simulink model "Sim_Riementrieb"  (R2015b)
settings: Solver=ode45  SolverMode=SingleTasking  StartTime=0.0  StopTime=10.0  RelTol=1e-3
undefined symbols (not defined in the file or in its folder): parSys
libraries: cstblocks x2
settings Model: Creator=wke  LastModifiedBy=danielhauer
settings DataIOCC: SaveFormat=Array  SignalLoggingSaveFormat=ModelDataLogs
settings OptimizationCC: BlockReduction=off  BooleanDataType=off
settings DebuggingCC: SaveWithParameterizedLinksMsg=none  UnderspecifiedInitializationDetection=Classic  MergeDetectMultiDrivingBlocksExec=none  SignalResolutionControl=TryResolveAllWithWarning  MultiTaskDSMMsg=warning  MultiTaskCondExecSysMsg=none  StateNameClashWarn=warning
settings HardwareCC: ProdBitPerPointer=32  ProdLargestAtomicFloat=None  ProdIntDivRoundTo=Undefined  ProdEndianess=Unspecified  ProdWordSize=32  ProdHWDeviceType=32-bit Generic  TargetUnknown=on
settings GRTTargetCC: GeneratePreprocessorConditionals=Disable all
settings ConfigComp: CovModelRefEnable=Off

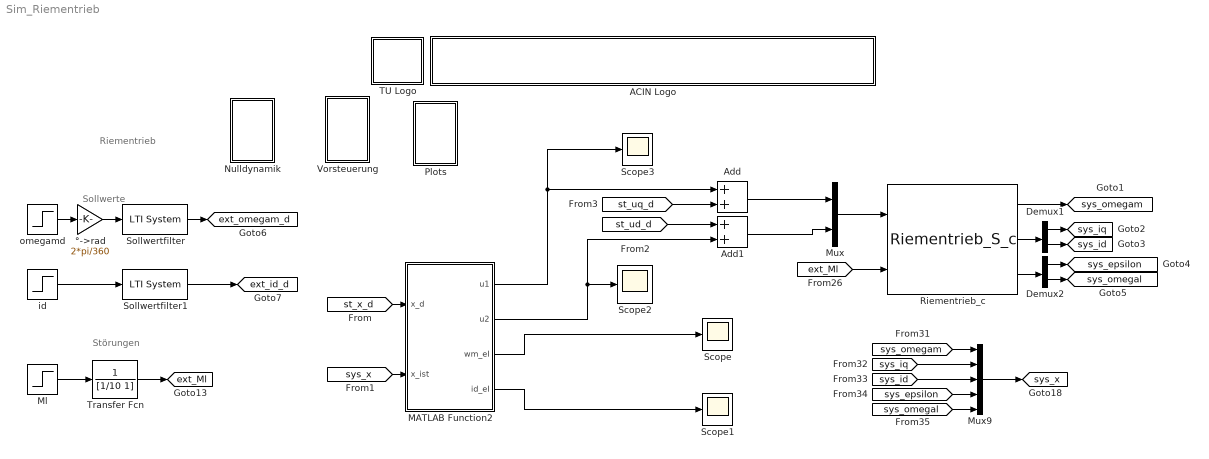
== system Sim_Riementrieb ==
  note: Riementrieb
  note: Sollwerte
  note: Störungen
  ACIN Logo : Subsystem
      mask init:
      | s = get_param(gcb,'UserData');
      mask Display:
      | image(s.logo,[0 0 439 45]);
      | %axis image
  Add : Sum
  Add1 : Sum
  Demux1 : Demux  Outputs=2
  Demux2 : Demux  Outputs=2
  MATLAB Function2 : MATLAB Function  TreatAsAtomicUnit=on  SystemSampleTime=parSys.TsID
  Ml : Step  Time=4  After=0.1  SampleTime=0
  Mux : Mux  Inputs=2
  Mux9 : Mux  Inputs=5
  Nulldynamik : Subsystem
  "Plots " : Subsystem
  Riementrieb_c : S-Function  FunctionName=Riementrieb_S_c  Parameters=parSys  SFunctionDeploymentMode=off  EnableBusSupport=off
      mask Display:
      | port_label('input',1,'uq,ud');
      | port_label('input',2,'Ml');
      | port_label('output',1,'omegam');
      | port_label('output',2,'iq,id');
      | port_label('output',3,'epsilon,omegal');
  Scope{,1..3} (4 alike) : Scope
  Sollwertfilter : cstblocks/LTI System  sys=parReg.ssSF  IC=[]
  Sollwertfilter1 : cstblocks/LTI System  sys=parReg.ssSFi  IC=[]
  TU Logo : Subsystem
      mask init:
      | s = get_param(gcb,'UserData');
      mask Display: image(s.logo,[0 0 45 45]);
  Transfer Fcn : TransferFcn  Denominator=[1/10 1]
  Vorsteuerung : Subsystem
  id : Step  Time=0.5  After=0.1  SampleTime=0
  omegamd : Step  Time=2  After=1000/60*360  SampleTime=0
  °->rad : Gain  Gain=2*pi/360
  tag scope: ext_Ml=global, ext_id_d=global, ext_omegam_d=global, sys_epsilon=global, sys_id=global, sys_iq=global, sys_omegal=global, sys_omegam=global, sys_x=global
  wires:
  Mux/1 -> Riementrieb_c/1
  °->rad/1 -> Sollwertfilter/1
  Sollwertfilter/1 -> [ext_omegam_d]
  Demux1/1 -> [sys_iq]
  Demux1/2 -> [sys_id]
  Demux2/1 -> [sys_epsilon]
  Demux2/2 -> [sys_omegal]
  Sollwertfilter1/1 -> [ext_id_d]
  id/1 -> Sollwertfilter1/1
  Ml/1 -> Transfer Fcn/1
  omegamd/1 -> °->rad/1
  Transfer Fcn/1 -> [ext_Ml]
  [ext_Ml] -> Riementrieb_c/2
  Riementrieb_c/2 -> Demux1/1
  Riementrieb_c/3 -> Demux2/1
  Riementrieb_c/1 -> [sys_omegam]
  [sys_omegam] -> Mux9/1
  [sys_iq] -> Mux9/2
  [sys_id] -> Mux9/3
  [sys_epsilon] -> Mux9/4
  [sys_omegal] -> Mux9/5
  Mux9/1 -> [sys_x]
  [st_x_d] -> MATLAB Function2/1(x_d)
  [sys_x] -> MATLAB Function2/2(x_ist)
  Add/1 -> Mux/1
  Add1/1 -> Mux/2
  MATLAB Function2/3(wm_eI) -> Scope/1
  MATLAB Function2/4(id_eI) -> Scope1/1
  [st_uq_d] -> Add/2
  [st_ud_d] -> Add1/1
  MATLAB Function2/1(u1) -> Scope3/1, Add/1
  MATLAB Function2/2(u2) -> Scope2/1, Add1/2

== system Sim_Riementrieb/ACIN Logo ==

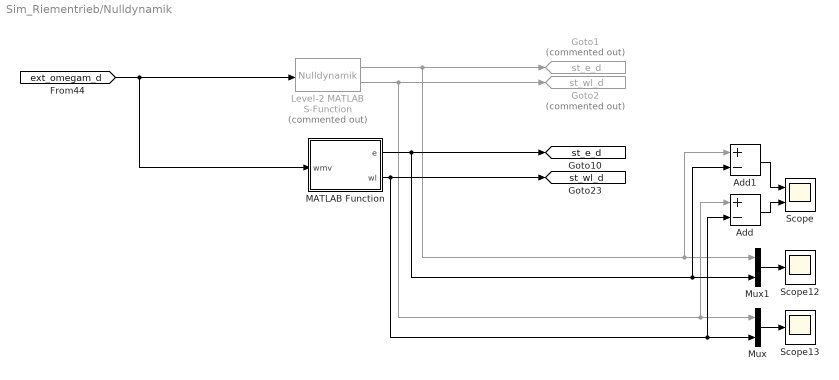
== system Sim_Riementrieb/Nulldynamik ==
  Add : Sum  Inputs=+-
  Add1 : Sum  Inputs=+-
  Goto1 : Goto  Commented=on  GotoTag=st_e_d  TagVisibility=global
  Goto2 : Goto  Commented=on  GotoTag=st_wl_d  TagVisibility=global
  Level-2 MATLAB S-Function : M-S-Function  Commented=on  FunctionName=Nulldynamik  Parameters=parSys.epsilon_0 parSys.omegal_0 [parSys.cr1 parSys.cr3 parSys.rl parSys.rm parSys.dl parSys.Il]
  MATLAB Function : MATLAB Function  TreatAsAtomicUnit=on
  Mux : Mux  Inputs=2
  Mux1 : Mux  Inputs=2
  Scope : Scope  NumInputPorts=2
  Scope12 : Scope
  Scope13 : Scope
  tag scope: st_e_d=global, st_wl_d=global
  wires:
  Level-2 MATLAB S-Function/1 -> Add1/1, Mux1/1, Goto1/1
  Level-2 MATLAB S-Function/2 -> Add/1, Mux/1, Goto2/1
  [ext_omegam_d] -> MATLAB Function/1(wmv), Level-2 MATLAB S-Function/1
  MATLAB Function/1(e) -> Add1/2, Mux1/2, [st_e_d]
  MATLAB Function/2(wl) -> Add/2, Mux/2, [st_wl_d]
  Mux/1 -> Scope13/1
  Mux1/1 -> Scope12/1
  Add/1 -> Scope/2
  Add1/1 -> Scope/1

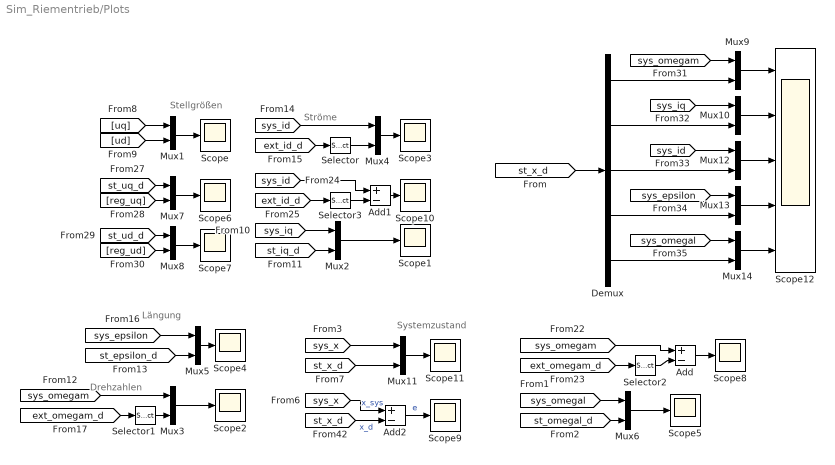
== system Sim_Riementrieb/Plots  ==
  note: Stellgrößen
  note: Ströme
  note: Drehzahlen
  note: Längung
  note: Systemzustand
  Add : Sum  Inputs=+-
  Add1 : Sum  Inputs=+-
  Add2 : Sum  Inputs=+-
  Demux : Demux  Outputs=5
  Mux{1..14} (14 alike) : Mux  Inputs=2
  Scope{,1..11} (12 alike) : Scope
  Scope12 : Scope  NumInputPorts=5
  Selector : Selector  InputPortWidth=2  IndexOptions=Index vector (dialog)  Indices=[1]  OutputSizes=1
  Selector1 : Selector  InputPortWidth=3  IndexOptions=Index vector (dialog)  Indices=[1]  OutputSizes=1
  Selector2 : Selector  InputPortWidth=3  IndexOptions=Index vector (dialog)  Indices=[1]  OutputSizes=1
  Selector3 : Selector  InputPortWidth=2  IndexOptions=Index vector (dialog)  Indices=[1]  OutputSizes=1
  wires:
  [uq] -> Mux1/1
  [ud] -> Mux1/2
  [sys_iq] -> Mux2/1
  Mux1/1 -> Scope/1
  Mux2/1 -> Scope1/1
  [st_iq_d] -> Mux2/2
  Mux3/1 -> Scope2/1
  [sys_omegam] -> Mux3/1
  [sys_epsilon] -> Mux5/1
  [sys_id] -> Mux4/1
  [ext_id_d] -> Selector/1
  Mux4/1 -> Scope3/1
  Mux5/1 -> Scope4/1
  [sys_omegal] -> Mux6/1
  [st_epsilon_d] -> Mux5/2
  Mux6/1 -> Scope5/1
  [ext_omegam_d] -> Selector1/1
  Selector1/1 -> Mux3/2
  Selector/1 -> Mux4/2
  [st_omegal_d] -> Mux6/2
  Add/1 -> Scope8/1
  [ext_omegam_d] -> Selector2/1
  [sys_omegam] -> Add/1
  [sys_id] -> Add1/1
  Selector2/1 -> Add/2
  Add1/1 -> Scope10/1
  [ext_id_d] -> Selector3/1
  Selector3/1 -> Add1/2
  [reg_uq] -> Mux7/2
  [st_uq_d] -> Mux7/1
  [st_ud_d] -> Mux8/1
  Mux7/1 -> Scope6/1
  [reg_ud] -> Mux8/2
  Mux8/1 -> Scope7/1
  Mux11/1 -> Scope11/1
  [sys_x] -> Mux11/1
  [st_x_d] -> Mux11/2
  [sys_x] -> Add2/1  "x_sys"
  Add2/1 -> Scope9/1  "e"
  [st_x_d] -> Add2/2  "x_d"
  [st_x_d] -> Demux/1
  Mux10/1 -> Scope12/2
  Mux12/1 -> Scope12/3
  Mux14/1 -> Scope12/5
  Demux/5 -> Mux14/2
  Demux/3 -> Mux12/2
  Demux/4 -> Mux13/2
  Demux/2 -> Mux10/2
  Demux/1 -> Mux9/2
  [sys_omegam] -> Mux9/1
  [sys_iq] -> Mux10/1
  [sys_id] -> Mux12/1
  [sys_epsilon] -> Mux13/1
  [sys_omegal] -> Mux14/1
  Mux13/1 -> Scope12/4
  Mux9/1 -> Scope12/1

== system Sim_Riementrieb/TU Logo ==

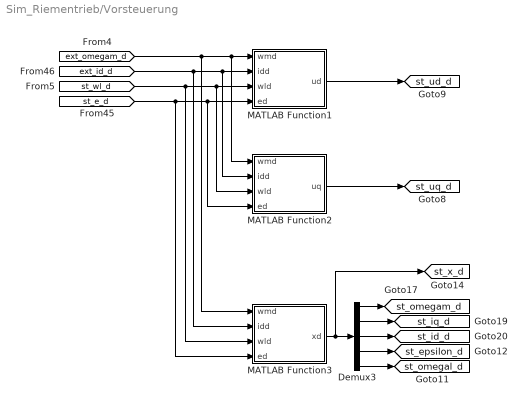
== system Sim_Riementrieb/Vorsteuerung ==
  Demux3 : Demux  Outputs=5
  MATLAB Function1 : MATLAB Function  TreatAsAtomicUnit=on
  MATLAB Function2 : MATLAB Function  TreatAsAtomicUnit=on
  MATLAB Function3 : MATLAB Function  TreatAsAtomicUnit=on
  tag scope: st_epsilon_d=global, st_id_d=global, st_iq_d=global, st_omegal_d=global, st_omegam_d=global, st_ud_d=global, st_uq_d=global, st_x_d=global
  wires:
  MATLAB Function2/1(uq) -> [st_uq_d]
  MATLAB Function3/1(xd) -> [st_x_d], Demux3/1
  Demux3/4 -> [st_epsilon_d]
  Demux3/5 -> [st_omegal_d]
  Demux3/1 -> [st_omegam_d]
  Demux3/2 -> [st_iq_d]
  Demux3/3 -> [st_id_d]
  [ext_omegam_d] -> MATLAB Function3/1(wmd), MATLAB Function2/1(wmd), MATLAB Function1/1(wmd)
  [st_wl_d] -> MATLAB Function3/3(wld), MATLAB Function2/3(wld), MATLAB Function1/3(wld)
  [st_e_d] -> MATLAB Function3/4(ed), MATLAB Function2/4(ed), MATLAB Function1/4(ed)
  MATLAB Function1/1(ud) -> [st_ud_d]
  [ext_id_d] -> MATLAB Function3/2(idd), MATLAB Function2/2(idd), MATLAB Function1/2(idd)

== matlab function Sim_Riementrieb/Vorsteuerung/MATLAB Function1 ==
  data: wmd input; idd input; ud output; wld input; ed input; parSys parameter
function ud  = fcn(wmd, idd, wld, ed, parSys)
%#codegen
wm = wmd(1);
wmp = wmd(2);
wmpp = wmd(3);
id = idd(1);
idp = idd(2);
wl = wld;
e = ed;

%parameter;
%Zuweisungen
Lm = parSys.Lm;
Rm = parSys.Rm;
cr1 = parSys.cr1;
cr3 = parSys.cr3;
rm = parSys.rm;
dm = parSys.dm;
rl = parSys.rl;
dl = parSys.dl;
I_l = parSys.Il;
I_m = parSys.Im;
p = parSys.p;
Phi = parSys.Phi;

iq = 0.2e1 / 0.3e1 * (-2 * cr3 * e ^ 3 * rm - 2 * cr1 * e * rm + wmp * I_m + dm * wm) / Phi / p;
ud = 0.3e1 / 0.2e1 * Lm * p * wm * iq + 0.3e1 / 0.2e1 * idp * Lm + Rm * id;


%ud = 3/2*Lm * (idp - 2/3*(-Rm*id - 3/2 * Lm * p * wm * iq)/Lm);

end

== matlab function Sim_Riementrieb/Nulldynamik/MATLAB Function ==
  settings: updateMethod=DISCRETE  sampleTime=parSys.TsID
  data: wmv input; e output; wl output; parSys parameter
function [e, wl] = Nulldynamik_diskret(wmv, parSys)
%#codegen
persistent k
persistent x1
persistent x2

wm = wmv(1);

if (isempty(k))
    k = 0;
end
if (isempty(x1))
    x1 = parSys.epsilon_0;
end
if (isempty(x2))
    x2 = parSys.omegal_0;
end

cr1 = parSys.cr1;
cr3 = parSys.cr3;
Il = parSys.Il;
rl = parSys.rl;
rm = parSys.rm;
dl = parSys.dl;

k = k + parSys.TsID;

f1 = rl*x2-rm*wm;
f2 = 1/Il*(-2*(cr1*x1+cr3*x1^3)*rl - dl*x2);

xp1 = x1 + parSys.TsID*f1;
xp2 = x2 + parSys.TsID*f2;

x1 = x1 + parSys.TsID/2*(f1 + (rl*xp2 - rm*wm));
x2  = x2 + parSys.TsID/2*(f2 + 1/Il*(-2*(cr1*xp1 + cr3*xp1^3)*rl - dl*xp2));

e = x1;
wl = x2;
end

== matlab function Sim_Riementrieb/Vorsteuerung/MATLAB Function2 ==
  data: wmd input; idd input; uq output; wld input; ed input; parSys parameter
function uq  = fcn(wmd, idd, wld, ed, parSys)
%#codegen
wm = wmd(1);
wmp = wmd(2);
wmpp = wmd(3);
id = idd(1);
idp = idd(2);
wl = wld;
e = ed;

%parameter;
%Zuweisungen
Lm = parSys.Lm;
Rm = parSys.Rm;
cr1 = parSys.cr1;
cr3 = parSys.cr3;
rm = parSys.rm;
dm = parSys.dm;
rl = parSys.rl;
dl = parSys.dl;
I_l = parSys.Il;
I_m = parSys.Im;
p = parSys.p;
Phi = parSys.Phi;

iq = 0.2e1 / 0.3e1 * (-2 * cr3 * e ^ 3 * rm - 2 * cr1 * e * rm + wmp * I_m + dm * wm) / Phi / p;
uq = Lm * I_m / Phi / p * (wmpp + 0.1e1 / I_m ^ 2 * dm * ((2 * (cr3 * e ^ 3 + cr1 * e) * rm) - dm * wm + 0.3e1 / 0.2e1 * Phi * p * iq) - 0.1e1 / I_m * Phi * p / Lm * (-Rm * iq + 0.3e1 / 0.2e1 * Lm * p * wm * id - Phi * p * wm) - 0.2e1 / I_m * (3 * cr3 * e ^ 2 + cr1) * rm * (rl * wl - rm * wm));


%ud = 3/2*Lm * (idp - 2/3*(-Rm*id - 3/2 * Lm * p * wm * iq)/Lm);

end

== matlab function Sim_Riementrieb/Vorsteuerung/MATLAB Function3 ==
  data: wmd input; idd input; xd output; wld input; ed input; parSys parameter
function xd  = fcn(wmd, idd, wld, ed, parSys)
%#codegen
wm = wmd(1);
wmp = wmd(2);
wmpp = wmd(3);
id = idd(1);
idp = idd(2);
wl = wld;
e = ed;

%parameter;
%Zuweisungen
Lm = parSys.Lm;
Rm = parSys.Rm;
cr1 = parSys.cr1;
cr3 = parSys.cr3;
rm = parSys.rm;
dm = parSys.dm;
rl = parSys.rl;
dl = parSys.dl;
I_l = parSys.Il;
I_m = parSys.Im;
p = parSys.p;
Phi = parSys.Phi;

iq = 0.2e1 / 0.3e1 * (-2 * cr3 * e ^ 3 * rm - 2 * cr1 * e * rm + wmp * I_m + dm * wm) / Phi / p;

xd = [wm iq id e wl];


end

== matlab function Sim_Riementrieb/MATLAB Function2 ==
  settings: updateMethod=DISCRETE  sampleTime=parSys.TsID
  data: x_d input; x_ist input; u1 output; u2 output; K parameter; wm_eI output; id_eI output
function [u1,u2,wm_eI,id_eI] = fcn(x_d,x_ist, K)
%#codegen

persistent t
persistent ewm_I
persistent eid_I
if (isempty(t))
   t = 0;
   ewm_I=0;
   eid_I=0;

end

ewm_I=ewm_I + 1e-4 *(x_ist(1)-x_d(1));
eid_I=eid_I + 1e-4 *(x_ist(3)-x_d(3));

wm_eI=ewm_I;
id_eI=eid_I;


t=t+1;


u=K(:,:,t)*[+x_ist-x_d';ewm_I;eid_I];

u1=u(1);
u2=u(2);

end
